simulink model "JKFF_Set"  (R2025b)
settings: Solver=VariableStepAuto  StartTime=0.0  StopTime=inf  FixedStep=0.01  RelTol=1e-3
libraries: simulink_extras x1
settings Model: PacingRate=1.100000  Creator=Soochan Kim  LastModifiedBy=Soochan Kim

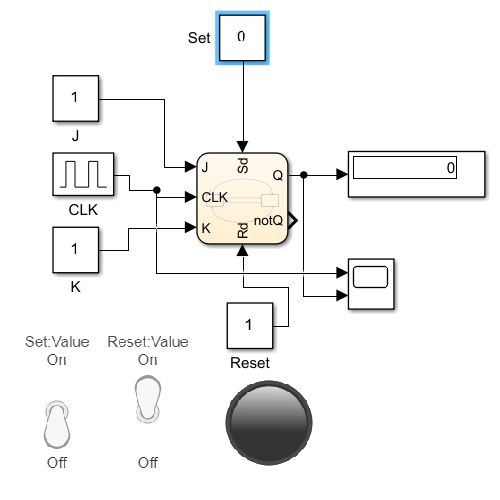
[thumbnail: Simulink's stored preview of the top-level diagram]
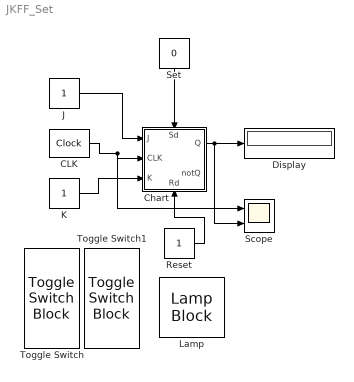
== system JKFF_Set ==
  CLK : simulink_extras/Flip Flops/Clock  period=2
  Chart : Stateflow chart  TreatAsAtomicUnit=on
      settings: PortSchema="{\"entries\":[{\"content\":{\"sides\":[{\"content\":{\"connectorIds\":[\"In1\",\"In2\",\"In3\"]},\"type\":\"ConnectorPlacement.EquallySpacedRectSide\",\"uuid\":\"2af75eb2-b907-44b2-82cc-b57e0a0d1c9b\"},{\"content\":{\"connectorIds\":[\"Out1\",\"Out2\"],\"side\":\"RIGHT\"},\"type\":\"ConnectorPlacement.EquallySpacedRectSide\",\"uuid\":\"6517b60d-825e-4e21-aa23-d5468b780dc3\"},{\"content\":{\"connectorIds\":[\"In4\"],\"side\":\"TOP\"},\"type\":\"ConnectorPlacement.EquallySpacedRectSide\",\"uuid\":\"6792e8eb-5222-4842-ba8a-bb88748afe2e\"},{\"content\":{\"connectorIds\":[\"In5\"],\"side\":\"BOTTOM\"},\"type\":\"ConnectorPlacement.EquallySpacedRectSide\",\"uuid\":\"cabb32ad-94a1-4a96-98a9-7356dbac5a93\"}]},\"type\":\"ConnectorPlacement.EquallySpacedConnector\",\"uuid\":\"0f8d812c-ded7-4acb-bdb8-74f44742dfe2\"}],\"packageUris\":[\"http://schema.mathworks.com/mf0/Connector/R2020b\"],\"version\":\"1.0\"}"
  Display : Display
  J : Constant
  K : Constant
  Lamp : LampBlock  LabelPosition=Hide  DefaultColor=[192.0, 192.0, 192.0]
  Reset : Constant
  Scope : Scope  NumInputPorts=2
      settings: SampleTime=0.1  ActiveDisplayYMinimum=-0.125  ActiveDisplayYMaximum=1.125
  Set : Constant  Value=0
  Toggle Switch : ToggleSwitchBlock
  Toggle Switch1 : ToggleSwitchBlock
  wires:
  J/1 -> Chart/1(J)
  K/1 -> Chart/3(K)
  CLK/1 -> Scope/1, Chart/2(CLK)
  Chart/1(Q) -> Scope/2, Display/1
  Set/1 -> Chart/4(Sd)
  Reset/1 -> Chart/5(Rd)

== stateflow chart JKFF_Set/Chart ==
  settings: updateMethod=DISCRETE  sampleTime=0.01
  state State_Q0
    entry:
    Q=0;
    notQ=1;
  state State_Q1
    entry:
    Q=1;
    notQ=0;
  State_Q0 -> State_Q1 [order 1] : [Sd==1 && Rd==0]
  (default) -> State_Q0
  State_Q0 -> State_Q1 [order 2] : [Rd == 0 && Sd == 0 && rising(CLK) && J==1]
  State_Q1 -> State_Q0 [order 2] : [Rd == 0 && Sd == 0 && rising(CLK) && K==1]
  State_Q1 -> State_Q0 [order 1] : [Rd==1]
  data: J input; Q output; CLK input; K input; Sd input; Rd input; notQ output
